simulink library "carnotUIBK"  (R2024b)
settings: Solver=VariableStepAuto  StartTime=0.0  StopTime=10.0  RelTol=1e-3  EnableMultiTasking=on
values from neighbouring files (symbols this model uses):
  area = area + room(kk).area    [THERMALZONE.m]
  boundary = BOUNDARY()    [BUILDING.m]
  building = obj    [BUILDING.m]
  C = zeros(1,length(d)+1)    [CONSTRUCTION.m]
  cp = str2num(value)    [CONSTRUCTION.m]
  pos = find(d_layer>0)    [CONSTRUCTION.m]
  rho = str2num(value)    [CONSTRUCTION.m]
  type = 1    [CONSTRUCTION.m]
  zone = obj.zone(ind)    [THERMALZONE.m]
undefined symbols (not defined in the file or in its folder): A, amb_factor, B, const, control, Dd, get_building, height, p, Qdot_C, Qdot_H, Qdot_I_electricity, Qdot_I_light, Qdot_I_person, Qdot_S, Qdot_T_ground, Qdot_T_neighbour, Qdot_T_opaque, Qdot_T_window, Qdot_V_infiltration, Qdot_V_mech, Qdot_V_window, r_frame, solar_ratio, solar_ratio1, solar_ratio2, Tc, Tr, Ts, Uvalue, view_factor, wall, wallsurface, window, window_height, window_heigth, window_width, windowsurface, x_CO2, x_H2O, x_VOC, z
libraries: carnot x105, $bdroot x22, simulink x18, simulink_extras x14
(part 3 of 13)

== system carnotUIBK/airexchange_intersection/EMPTY ==
  AIB1 : Inport
  AIB2 : Inport  Port=2
  control : Inport  Port=3
  Constant{,1..12,17..19} (16 alike) : Constant  Value=0
  Constant13 : Constant  Value=zeros(1,6)
  Constant14 : Constant  Value=zeros(1,5)
  Constant15 : Constant  Value=zeros(1,6)
  Constant16 : Constant  Value=zeros(1,5)
  Mux1 : Mux  Inputs=[1 1 1 1 1 1 1 6 1 5]
  Mux2 : Mux  Inputs=[1 1 1 1 1 1 1 6 1 5]
  Selector1 : Selector  InputPortWidth=NUMBEROFCONTROLS  IndexOptions=Index vector (dialog)  Indices=[control]  OutputSizes=1
  Terminator : Terminator
  Terminator1 : Terminator
  Terminator2 : Terminator
  "[S1]" : Outport  InitialOutput=0  VectorParamsAs1DForOutWhenUnconnected=off
  "[S2]" : Outport  Port=2  InitialOutput=0  VectorParamsAs1DForOutWhenUnconnected=off
  wires:
  Constant1/1 -> Mux1/4
  Constant4/1 -> Mux1/9
  Constant3/1 -> Mux1/6
  Constant2/1 -> Mux1/5
  Constant/1 -> Mux1/1
  Mux1/1 -> "[S1]"/1
  AIB2/1 -> Terminator2/1
  AIB1/1 -> Terminator1/1
  Constant11/1 -> Mux1/3
  Constant10/1 -> Mux1/2
  Constant12/1 -> Mux1/7
  Constant13/1 -> Mux1/8
  Constant14/1 -> Mux1/10
  control/1 -> Selector1/1
  Selector1/1 -> Terminator/1
  Mux2/1 -> "[S2]"/1
  Constant6/1 -> Mux2/4
  Constant19/1 -> Mux2/9
  Constant18/1 -> Mux2/6
  Constant17/1 -> Mux2/5
  Constant5/1 -> Mux2/1
  Constant8/1 -> Mux2/3
  Constant7/1 -> Mux2/2
  Constant9/1 -> Mux2/7
  Constant15/1 -> Mux2/8
  Constant16/1 -> Mux2/10

== system carnotUIBK/airexchange_intersection/airexchange_empiric ==
  note: ASSUMPTION: mdot_air_in = mdot_air_out !
  AIB1 : Inport
  AIB2 : Inport  Port=2
  control : Inport  Port=3
  1/3600 : Gain  Gain=1/3600
  Bus Selector1 : BusSelector  OutputSignals=Tc,x_H2O,x_CO2
  Bus Selector2 : BusSelector  OutputSignals=Tc,x_H2O,x_CO2,rho,cp
  Constant{4..6,9,15..16} (6 alike) : Constant  Value=0
  Constant17 : Constant  Value=zeros(1,2)
  Constant18 : Constant  Value=zeros(1,9)
  Constant7 : Constant  Value=zeros(1,2)
  Constant8 : Constant  Value=zeros(1,9)
  Gain{1,4..6} (4 alike) : Gain  Gain=-1
  Gain2 : Gain  Gain=0
  Gain3 : Gain  Gain=0
  Mux : Mux  Inputs=2
  Mux1 : Mux  Inputs=[1 1 1 1 1 1 1 2 1 9]
  Mux2 : Mux  Inputs=[1 1 1 1 1 1 1 2 1 9]
  Mux3 : Mux  Inputs=2
  Product2 : Product  InputSameDT=on  SaturateOnIntegerOverflow=on  OutDataTypeStr=Inherit: Same as first input
  Product4 : Product  Inputs=3  InputSameDT=on  SaturateOnIntegerOverflow=on  OutDataTypeStr=Inherit: Same as first input
  Selector1 : Selector  InputPortWidth=NUMBEROFCONTROLS  IndexOptions=Index vector (dialog)  Indices=[control]  OutputSizes=1
  Subsystem : Subsystem
  Sum : Sum  Inputs=-+  InputSameDT=on  SaturateOnIntegerOverflow=on  OutDataTypeStr=Inherit: Same as first input
  V exchange : Subsystem
  "[S1]" : Outport  InitialOutput=0  VectorParamsAs1DForOutWhenUnconnected=off
  "[S2]" : Outport  Port=2  InitialOutput=0  VectorParamsAs1DForOutWhenUnconnected=off
  wires:
  Gain2/1 -> Mux1/4
  Sum/1 -> Product4/1  "dT"
  Bus Selector2/5 -> Product4/2  "<cp>"
  Mux1/1 -> "[S1]"/1
  Bus Selector2/3 -> Mux/2  "<x_CO2>"
  control/1 -> Selector1/1
  AIB1/1 -> Bus Selector2/1
  AIB2/1 -> Bus Selector1/1
  Bus Selector2/4 -> Product2/2  "<rho>"
  Product4/1 -> Gain4/1, Gain1/1, Mux1/9, Mux1/1  "Qdot_air"
  Subsystem/2(mdot_CO2) -> Mux1/6, Gain6/1  "mdot_CO2"
  Subsystem/1(mdot_H2O) -> Gain5/1, Mux1/5  "mdot_H2O"
  Bus Selector2/2 -> V exchange/2(x in), Mux/1  "<x_H2O>"
  Mux/1 -> Subsystem/2(x_in)
  Mux3/1 -> Subsystem/3(x_out)
  Selector1/1 -> V exchange/5(control)
  Mux2/1 -> "[S2]"/1
  Bus Selector1/2 -> V exchange/4(x out), Mux3/1  "<x_H2O>"
  Bus Selector1/3 -> Mux3/2  "<x_CO2>"
  V exchange/1(V exchange) -> 1/3600/1
  Bus Selector1/1 -> Sum/2, V exchange/3(Tc out)  "<Tc>"
  Bus Selector2/1 -> Sum/1, V exchange/1(Tc in)  "<Tc>"
  1/3600/1 -> Product2/1
  Product2/1 -> Product4/3, Subsystem/1(mdot_air), Gain2/1, Gain3/1
  Constant5/1 -> Mux1/3
  Constant4/1 -> Mux1/2
  Constant6/1 -> Mux1/7
  Constant7/1 -> Mux1/8
  Constant8/1 -> Mux1/10
  Constant15/1 -> Mux2/3
  Constant9/1 -> Mux2/2
  Constant16/1 -> Mux2/7
  Constant17/1 -> Mux2/8
  Constant18/1 -> Mux2/10
  Gain1/1 -> Mux2/9
  Gain3/1 -> Mux2/4
  Gain4/1 -> Mux2/1
  Gain5/1 -> Mux2/5
  Gain6/1 -> Mux2/6

== system carnotUIBK/airexchange_intersection/airexchange_powerlaw ==
  note: ASSUMPTION: mdot_air_in = mdot_air_out !
  AIB1 : Inport
  AIB2 : Inport  Port=2
  control : Inport  Port=3
  Bus Selector2 : BusSelector  OutputSignals=Tc,x_H2O,x_CO2,rho
  Bus Selector3 : BusSelector  OutputSignals=Tc,x_H2O,x_CO2,rho,cp
  Constant{4..6,9,15..16} (6 alike) : Constant  Value=0
  Constant17 : Constant  Value=zeros(1,2)
  Constant18 : Constant  Value=zeros(1,9)
  Constant7 : Constant  Value=zeros(1,2)
  Constant8 : Constant  Value=zeros(1,9)
  Divide1 : Product  Inputs=*/
  Gain{1,4..6} (4 alike) : Gain  Gain=-1
  Gain2 : Gain  Gain=0
  Gain3 : Gain  Gain=0
  Mux : Mux  Inputs=2
  Mux1 : Mux  Inputs=[1 1 1 1 1 1 1 2 1 9]
  Mux2 : Mux  Inputs=[1 1 1 1 1 1 1 2 1 9]
  Mux3 : Mux  Inputs=2
  Product4 : Product  Inputs=3  InputSameDT=on  SaturateOnIntegerOverflow=on  OutDataTypeStr=Inherit: Same as first input
  Selector1 : Selector  InputPortWidth=NUMBEROFCONTROLS  IndexOptions=Index vector (dialog)  Indices=[control]  OutputSizes=1
  Subsystem : Subsystem
  Sum : Sum  Inputs=-+  InputSameDT=on  SaturateOnIntegerOverflow=on  OutDataTypeStr=Inherit: Same as first input
  Transfer Fcn : TransferFcn  Denominator=[100 1]
  door open : Subsystem
  "door_area " : Constant  Value=area
  door_height : Constant  Value=height
  "door_height " : Constant  Value=height
  "[S1]" : Outport  InitialOutput=0  VectorParamsAs1DForOutWhenUnconnected=off
  "[S2]" : Outport  Port=2  InitialOutput=0  VectorParamsAs1DForOutWhenUnconnected=off
  wires:
  Gain2/1 -> Mux1/4
  Sum/1 -> Product4/1  "dT"
  Bus Selector3/5 -> Product4/2  "<cp>"
  Mux1/1 -> "[S1]"/1
  Bus Selector3/3 -> Mux/2  "<x_CO2>"
  control/1 -> Selector1/1
  AIB1/1 -> Bus Selector3/1
  AIB2/1 -> Bus Selector2/1
  Bus Selector2/1 -> Sum/2  "<Tc>"
  Bus Selector3/2 -> Mux/1  "<x_H2O>"
  Mux/1 -> Subsystem/2(x_in)
  Bus Selector3/1 -> Sum/1  "<Tc>"
  Mux3/1 -> Subsystem/3(x_out)
  Selector1/1 -> door open/5(control)
  door open/1(m_dot_open_door) -> Transfer Fcn/1
  Mux2/1 -> "[S2]"/1
  Product4/1 -> Gain6/1, Gain1/1, Mux1/9, Mux1/1  "Qdot_air"
  Subsystem/2(mdot_CO2) -> Gain4/1, Mux1/6  "mdot_CO2"
  Subsystem/1(mdot_H2O) -> Gain5/1, Mux1/5  "mdot_H2O"
  Bus Selector2/2 -> Mux3/1  "<x_H2O>"
  Bus Selector2/3 -> Mux3/2  "<x_CO2>"
  door_height/1 -> door open/1(H (height of the door [m]))
  Divide1/1 -> door open/4(L)  "door width"
  Bus Selector3/4 -> door open/2(rho_i)  "<rho>"
  Bus Selector2/4 -> door open/3(rho_j)  "<rho>"
  "door_area "/1 -> Divide1/1
  "door_height "/1 -> Divide1/2
  Constant5/1 -> Mux1/3
  Constant4/1 -> Mux1/2
  Constant6/1 -> Mux1/7
  Constant7/1 -> Mux1/8
  Constant8/1 -> Mux1/10
  Constant15/1 -> Mux2/3
  Constant9/1 -> Mux2/2
  Constant16/1 -> Mux2/7
  Constant17/1 -> Mux2/8
  Constant18/1 -> Mux2/10
  Gain1/1 -> Mux2/9
  Gain3/1 -> Mux2/4
  Gain4/1 -> Mux2/6
  Gain5/1 -> Mux2/5
  Gain6/1 -> Mux2/1
  Transfer Fcn/1 -> Gain3/1, Gain2/1, Subsystem/1(mdot_air), Product4/3

== system carnotUIBK/boundary/GDB ==
  GDB_create : BusCreator  Inputs=6
  ground_1 : FromWorkspace  VariableName=b.boundary.ground(1).temperature
  ground_2 : FromWorkspace  VariableName=b.boundary.ground(2).temperature
  ground_3 : FromWorkspace  VariableName=b.boundary.ground(3).temperature
  ground_4 : FromWorkspace  VariableName=b.boundary.ground(4).temperature
  ground_5 : FromWorkspace  VariableName=b.boundary.ground(5).temperature
  ground_6 : FromWorkspace  VariableName=b.boundary.ground(6).temperature
  GDB : Outport  VectorParamsAs1DForOutWhenUnconnected=off
  wires:
  ground_1/1 -> GDB_create/1  "ground_1"
  ground_3/1 -> GDB_create/3  "ground_3"
  ground_2/1 -> GDB_create/2  "ground_2"
  ground_6/1 -> GDB_create/6  "ground_6"
  ground_4/1 -> GDB_create/4  "ground_4"
  GDB_create/1 -> GDB/1
  ground_5/1 -> GDB_create/5  "ground_5"

== system carnotUIBK/boundary/NDB ==
  GDB_create : BusCreator  Inputs=6
  neighbour_1 : FromWorkspace  VariableName=b.boundary.neighbour(1).temperature
  neighbour_2 : FromWorkspace  VariableName=b.boundary.neighbour(2).temperature
  neighbour_3 : FromWorkspace  VariableName=b.boundary.neighbour(3).temperature
  neighbour_4 : FromWorkspace  VariableName=b.boundary.neighbour(4).temperature
  neighbour_5 : FromWorkspace  VariableName=b.boundary.neighbour(5).temperature
  neighbour_6 : FromWorkspace  VariableName=b.boundary.neighbour(6).temperature
  NDB : Outport  VectorParamsAs1DForOutWhenUnconnected=off
  wires:
  neighbour_5/1 -> GDB_create/5  "neighbour_5"
  GDB_create/1 -> NDB/1
  neighbour_4/1 -> GDB_create/4  "neighbour_4"
  neighbour_6/1 -> GDB_create/6  "neighbour_6"
  neighbour_2/1 -> GDB_create/2  "neighbour_2"
  neighbour_3/1 -> GDB_create/3  "neighbour_3"
  neighbour_1/1 -> GDB_create/1  "neighbour_1"

== system carnotUIBK/boundary/WDB ==
  I_diffuse_surface : FromWorkspace  VariableName=we.Idiffuse_surface
  I_direct_surface : FromWorkspace  VariableName=we.Idirect_surface
  WDB_Creator : carnot/Basic/Weather_and_Sun/WDB_Creator
      settings: SourceProductName=Carnot
  azimuth : FromWorkspace  VariableName=we.azimuth
  cloud_index : FromWorkspace  VariableName=we.cloud
  incidence : FromWorkspace  VariableName=we.incidence
  precipitation : FromWorkspace  VariableName=we.precip
  pressure : FromWorkspace  VariableName=we.p
  radiation_beam_normal : FromWorkspace  VariableName=we.radiation_beam_normal
  radiation_diffuse_horizontal : FromWorkspace  VariableName=we.radiation_diffuse_horizontal
  relative_humidity : FromWorkspace  VariableName=we.rh
  t_amb : FromWorkspace  VariableName=we.t_ambient
  t_sky : FromWorkspace  VariableName=we.t_sky
  teta_p : FromWorkspace  VariableName=we.tetap
  teta_s : FromWorkspace  VariableName=we.tetas
  time_value : FromWorkspace  VariableName=we.time_value
  vw : FromWorkspace  VariableName=we.vw
  wdir : FromWorkspace  VariableName=we.wdir
  zenith : FromWorkspace  VariableName=we.zenith
  WDB : Outport  VectorParamsAs1DForOutWhenUnconnected=off
  wires:
  radiation_beam_normal/1 -> WDB_Creator/4  "I_beam_normal"
  azimuth/1 -> WDB_Creator/3  "azimuth"
  t_amb/1 -> WDB_Creator/6  "Tamb"
  radiation_diffuse_horizontal/1 -> WDB_Creator/5  "I_diffuse_horizontal"
  time_value/1 -> WDB_Creator/1  "time_value"
  zenith/1 -> WDB_Creator/2  "zenith"
  t_sky/1 -> WDB_Creator/7  "Tsky"
  teta_p/1 -> WDB_Creator/15  "longitudinal_angle"
  relative_humidity/1 -> WDB_Creator/8  "relative_humidity"
  precipitation/1 -> WDB_Creator/9  "precipitation"
  cloud_index/1 -> WDB_Creator/10  "cloud_index"
  I_diffuse_surface/1 -> WDB_Creator/18  "I_diffuse_surface"
  pressure/1 -> WDB_Creator/11  "pressure"
  wdir/1 -> WDB_Creator/13  "wind_direction"
  teta_s/1 -> WDB_Creator/16  "transversal_angle"
  I_direct_surface/1 -> WDB_Creator/17  "I_direct_surface"
  vw/1 -> WDB_Creator/12  "wind_speed"
  incidence/1 -> WDB_Creator/14  "incidence_angle"
  WDB_Creator/1 -> WDB/1

== system carnotUIBK/gain/EMPTY ==
  AIB : Inport
  control : Inport  Port=2
  Constant13 : Constant  Value=zeros(1,19)
  Mux1 : Mux  Inputs=[19]
  Selector1 : Selector  InputPortWidth=NUMBEROFCONTROLS  IndexOptions=Index vector (dialog)  Indices=[control]  OutputSizes=1
  Terminator : Terminator
  Terminator1 : Terminator
  "[S]" : Outport  VectorParamsAs1DForOutWhenUnconnected=off
  wires:
  AIB/1 -> Terminator/1
  Mux1/1 -> "[S]"/1
  control/1 -> Selector1/1
  Selector1/1 -> Terminator1/1
  Constant13/1 -> Mux1/1

== system carnotUIBK/gain/Equipment ==
  AIB : Inport
  control : Inport  Port=2
  0 : Constant  Value=0
  1 : Constant
  Product : Product
  Selector1 : Selector  InputPortWidth=NUMBEROFCONTROLS  IndexOptions=Index vector (dialog)  Indices=[control]  OutputSizes=1
  Sum : Sum  Inputs=|+-
  Sum1 : Sum  InputSameDT=on  SaturateOnIntegerOverflow=on  OutDataTypeStr=Inherit: Same as first input
  Sum2 : Sum  Inputs=|+-
  Switch : Constant  Value=type
  Switch1 : Switch  Criteria=u2 ~= 0  SaturateOnIntegerOverflow=off  InputSameDT=off
  Switch2 : Switch  Criteria=u2 ~= 0  SaturateOnIntegerOverflow=off  InputSameDT=off
  Terminator : Terminator
  W/device : Subsystem
  W/m² : Subsystem
  none : Constant  Value=0
  none1 : Constant  Value=0
  okay : Constant
  okay1 : Constant
  "[S]" : Outport  VectorParamsAs1DForOutWhenUnconnected=off
  wires:
  W/m²/1("[S]") -> Sum1/2
  W/device/1("[S]") -> Sum1/1
  Switch/1 -> Sum/1, Sum2/1
  0/1 -> Sum/2
  Sum/1 -> Switch1/2
  okay/1 -> Switch1/3
  none/1 -> Switch1/1
  1/1 -> Sum2/2
  Sum2/1 -> Switch2/2
  okay1/1 -> Switch2/3
  none1/1 -> Switch2/1
  Switch1/1 -> W/device/1(Switch)
  Switch2/1 -> W/m²/1(Switch)
  AIB/1 -> Terminator/1
  control/1 -> Selector1/1
  Selector1/1 -> Product/2
  Product/1 -> "[S]"/1
  Sum1/1 -> Product/1

== system carnotUIBK/gain/Light ==
  AIB : Inport
  control : Inport  Port=2
  0 : Constant  Value=0
  1 : Constant
  Product : Product
  Selector1 : Selector  InputPortWidth=NUMBEROFCONTROLS  IndexOptions=Index vector (dialog)  Indices=[control]  OutputSizes=1
  Sum : Sum  Inputs=|+-
  Sum1 : Sum  InputSameDT=on  SaturateOnIntegerOverflow=on  OutDataTypeStr=Inherit: Same as first input
  Sum2 : Sum  Inputs=|+-
  Switch : Constant  Value=type
  Switch1 : Switch  Criteria=u2 ~= 0  SaturateOnIntegerOverflow=off  InputSameDT=off
  Switch2 : Switch  Criteria=u2 ~= 0  SaturateOnIntegerOverflow=off  InputSameDT=off
  Terminator : Terminator
  W/light : Subsystem
  W/m² : Subsystem
  none : Constant  Value=0
  none1 : Constant  Value=0
  okay : Constant
  okay1 : Constant
  "[S]" : Outport  VectorParamsAs1DForOutWhenUnconnected=off
  wires:
  W/m²/1("[S]") -> Sum1/2
  W/light/1("[S]") -> Sum1/1
  AIB/1 -> Terminator/1
  ? -> ?
  Switch/1 -> Sum/1, Sum2/1
  0/1 -> Sum/2
  Sum/1 -> Switch1/2
  okay/1 -> Switch1/3
  none/1 -> Switch1/1
  1/1 -> Sum2/2
  Sum2/1 -> Switch2/2
  okay1/1 -> Switch2/3
  none1/1 -> Switch2/1
  Switch1/1 -> W/light/1(Switch)
  Switch2/1 -> W/m²/1(Switch)
  control/1 -> Selector1/1
  Selector1/1 -> Product/2
  Product/1 -> "[S]"/1
  Sum1/1 -> Product/1

== system carnotUIBK/gain/Moisture ==
  AIB : Inport
  control : Inport  Port=2
  Product : Product
  Selector1 : Selector  InputPortWidth=NUMBEROFCONTROLS  IndexOptions=Index vector (dialog)  Indices=[control]  OutputSizes=1
  Terminator : Terminator
  kg/s : Subsystem
  "[S]" : Outport  VectorParamsAs1DForOutWhenUnconnected=off
  wires:
  AIB/1 -> Terminator/1
  control/1 -> Selector1/1
  Selector1/1 -> Product/2
  Product/1 -> "[S]"/1
  kg/s/1("[S]") -> Product/1

== system carnotUIBK/gain/People ==
  AIB : Inport
  control : Inport  Port=2
  0 : Constant  Value=0
  1 : Constant
  2 : Constant  Value=2
  Bus Selector : BusSelector  OutputSignals=Ts
  Constant : Constant  Value=type
  Product : Product
  Selector1 : Selector  InputPortWidth=NUMBEROFCONTROLS  IndexOptions=Index vector (dialog)  Indices=[control]  OutputSizes=1
  Sum : Sum  Inputs=|+-
  Sum1 : Sum  Inputs=+++  InputSameDT=on  SaturateOnIntegerOverflow=on  OutDataTypeStr=Inherit: Same as first input
  Sum2 : Sum  Inputs=|+-
  Sum3 : Sum  Inputs=|+-
  Switch : Switch  Criteria=u2 ~= 0  SaturateOnIntegerOverflow=off  InputSameDT=off
  Switch1 : Switch  Criteria=u2 ~= 0  SaturateOnIntegerOverflow=off  InputSameDT=off
  Switch2 : Switch  Criteria=u2 ~= 0  SaturateOnIntegerOverflow=off  InputSameDT=off
  W/m² : Subsystem
  W/ppl (activity) : Subsystem
  W/ppl (constant) : Subsystem
  none : Constant  Value=0
  none1 : Constant  Value=0
  none2 : Constant  Value=0
  okay : Constant
  okay1 : Constant
  okay2 : Constant
  "[S]" : Outport  VectorParamsAs1DForOutWhenUnconnected=off
  wires:
  W/m²/1("[S]") -> Sum1/3
  W/ppl (constant)/1("[S]") -> Sum1/1
  W/ppl (activity)/1("[S]") -> Sum1/2
  Constant/1 -> Sum/1, Sum2/1, Sum3/1
  0/1 -> Sum/2
  Sum/1 -> Switch/2
  okay/1 -> Switch/3
  none/1 -> Switch/1
  Switch/1 -> W/ppl (constant)/2(Switch)
  1/1 -> Sum2/2
  Sum2/1 -> Switch1/2
  Sum3/1 -> Switch2/2
  2/1 -> Sum3/2
  Switch1/1 -> W/ppl (activity)/2(Switch)
  Switch2/1 -> W/m²/1(Switch)
  okay1/1 -> Switch1/3
  none1/1 -> Switch1/1
  okay2/1 -> Switch2/3
  none2/1 -> Switch2/1
  AIB/1 -> Bus Selector/1
  Bus Selector/1 -> W/ppl (activity)/1(Top), W/ppl (constant)/1(Top)  "<Ts>"
  control/1 -> Selector1/1
  Selector1/1 -> Product/2
  Product/1 -> "[S]"/1
  Sum1/1 -> Product/1

== system carnotUIBK/general/S_initialize ==
  Bus Creator2 : BusCreator  Inputs=19
  Constant{,1..18} (19 alike) : Constant  Value=0
  S : Outport  VectorParamsAs1DForOutWhenUnconnected=off
  wires:
  Constant7/1 -> Bus Creator2/15  "Qdot_I_person"
  Constant11/1 -> Bus Creator2/18  "Qdot_H"
  Constant10/1 -> Bus Creator2/17  "Qdot_I_electricity"
  Constant9/1 -> Bus Creator2/16  "Qdot_I_light"
  Constant12/1 -> Bus Creator2/19  "Qdot_C"
  Bus Creator2/1 -> S/1
  Constant1/1 -> Bus Creator2/2  "Qdotr"
  Constant/1 -> Bus Creator2/1  "Qdotc"
  Constant8/1 -> Bus Creator2/3  "Qdot_S"
  Constant14/1 -> Bus Creator2/5  "mdot_H2O"
  Constant13/1 -> Bus Creator2/4  "mdot_air"
  Constant15/1 -> Bus Creator2/6  "mdot_CO2"
  Constant16/1 -> Bus Creator2/7  "mdot_VOC"
  Constant17/1 -> Bus Creator2/8  "Qdot_T_opaque"
  Constant5/1 -> Bus Creator2/13  "Qdot_V_window"
  Constant4/1 -> Bus Creator2/12  "Qdot_V_mech"
  Constant2/1 -> Bus Creator2/10  "Qdot_T_neighbour"
  Constant6/1 -> Bus Creator2/14  "Qdot_V_infiltration"
  Constant3/1 -> Bus Creator2/11  "Qdot_T_window"
  Constant18/1 -> Bus Creator2/9  "Qdot_T_ground"

== system carnotUIBK/general/density and capacity ==
  T : Inport
  p : Inport  Port=2
  Add : Sum  Inputs=2
  Constant1 : Constant  Value=10000
  Constant2 : Constant  Value=0.0001
  Divide : Product  Inputs=*/
  K : Constant  Value=273.15
  Product : Product
  Product1 : Product
  Ra : Gain  Gain=287.058
  Rounding Function : Rounding
  cp_const : Constant  Value=1006.8
  rho : Outport  VectorParamsAs1DForOutWhenUnconnected=off
  cp : Outport  Port=2  VectorParamsAs1DForOutWhenUnconnected=off
  wires:
  Product1/1 -> rho/1
  Constant2/1 -> Product1/2
  Constant1/1 -> Product/2
  Product/1 -> Rounding Function/1
  Divide/1 -> Product/1
  Rounding Function/1 -> Product1/1
  Ra/1 -> Divide/2
  Add/1 -> Ra/1
  K/1 -> Add/2
  T/1 -> Add/1
  p/1 -> Divide/1
  cp_const/1 -> cp/1

== system carnotUIBK/infiltration/EMPTY ==
  AIB : Inport
  WDB : Inport  Port=2
  control : Inport  Port=3
  Constant{,1..4,10..12} (8 alike) : Constant  Value=0
  Constant13 : Constant  Value=zeros(1,6)
  Constant14 : Constant  Value=zeros(1,5)
  Mux1 : Mux  Inputs=[1 1 1 1 1 1 1 6 1 5]
  Selector1 : Selector  InputPortWidth=NUMBEROFCONTROLS  IndexOptions=Index vector (dialog)  Indices=[control]  OutputSizes=1
  Terminator : Terminator
  Terminator1 : Terminator
  Terminator2 : Terminator
  "[S]" : Outport  InitialOutput=0  VectorParamsAs1DForOutWhenUnconnected=off
  wires:
  Selector1/1 -> Terminator/1
  control/1 -> Selector1/1
  AIB/1 -> Terminator1/1
  WDB/1 -> Terminator2/1
  Mux1/1 -> "[S]"/1
  Constant1/1 -> Mux1/4
  Constant4/1 -> Mux1/9
  Constant3/1 -> Mux1/6
  Constant2/1 -> Mux1/5
  Constant/1 -> Mux1/1
  Constant11/1 -> Mux1/3
  Constant10/1 -> Mux1/2
  Constant12/1 -> Mux1/7
  Constant13/1 -> Mux1/8
  Constant14/1 -> Mux1/10

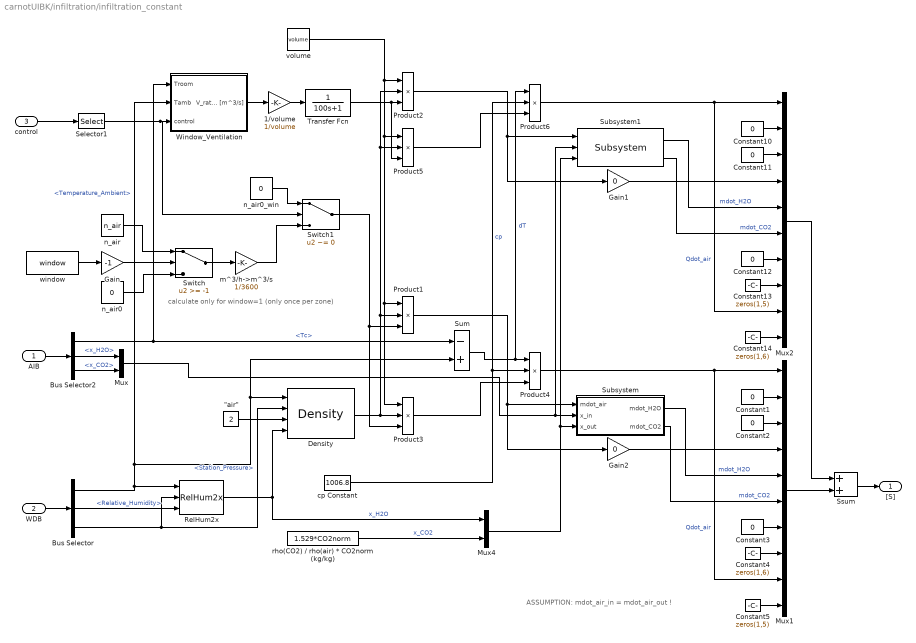
== system carnotUIBK/infiltration/infiltration_constant ==
  note: calculate only for window=1 (only once per zone)
  note: ASSUMPTION: mdot_air_in = mdot_air_out !
  AIB : Inport
  WDB : Inport  Port=2
  control : Inport  Port=3
  "\"air\"" : Constant  Value=2
  1/volume : Gain  Gain=1/volume
  Bus Selector : BusSelector  OutputSignals=Temperature_Ambient,Relative_Humidity,Station_Pressure
  Bus Selector2 : BusSelector  OutputSignals=Tc,x_H2O,x_CO2
  Constant{1..3,10..12} (6 alike) : Constant  Value=0
  Constant13 : Constant  Value=zeros(1,5)
  Constant14 : Constant  Value=zeros(1,6)
  Constant4 : Constant  Value=zeros(1,6)
  Constant5 : Constant  Value=zeros(1,5)
  Density : carnot/Basic/Material_Properties/Density  VariantControl=CarlibClassic  INPUTARGUMENTS=state variables (classic)  DEBUGLEVEL=NOLEVEL  MAXTOTALWARNINGS=inf  MAXCONSECUTIVEWARNINGS=inf  WRITETOFILE=0  FILENAME='errors.txt'
      settings: SourceProductName=Carnot
  Gain : Gain  Gain=-1
  Gain1 : Gain  Gain=0
  Gain2 : Gain  Gain=0
  Mux : Mux  Inputs=2
  Mux1 : Mux  Inputs=[1 1 1 1 1 1 1 6 1 5]
  Mux2 : Mux  Inputs=[1 1 1 1 1 1 1 5 1 6]
  Mux4 : Mux  Inputs=2
  Product{1..6} (6 alike) : Product  Inputs=3  InputSameDT=on  SaturateOnIntegerOverflow=on  OutDataTypeStr=Inherit: Same as first input
  RelHum2x : carnot/Basic/Material_Properties/RelHum2x
      settings: SourceProductName=Carnot
  Selector1 : Selector  InputPortWidth=NUMBEROFCONTROLS  IndexOptions=Index vector (dialog)  Indices=[control]  OutputSizes=1
  Ssum : Sum
  Subsystem : Subsystem
  Subsystem1 : $bdroot/infiltration/infiltration_constant/Subsystem  SystemSampleTime=-1  Latency=0  AutoFrameSizeCalculation=off
  Sum : Sum  Inputs=-+  InputSameDT=on  SaturateOnIntegerOverflow=on  OutDataTypeStr=Inherit: Same as first input
  Switch : Switch  Threshold=-1  SaturateOnIntegerOverflow=off  InputSameDT=off
  Switch1 : Switch  Criteria=u2 ~= 0  Threshold=-1  SaturateOnIntegerOverflow=off  InputSameDT=off
  Transfer Fcn : TransferFcn  Denominator=[100 1]
  Window_Ventilation : Subsystem  mask(window ventilation){alpha=10, H=window_width, W=window_height}
      mask prompts: alpha "maximal opening angle (°)"; H "height of window (m)"; W "width of window (m)"
      mask help: Simulates the free driven ventilation through a window with an opening angle of [0,1]* max. angle. Valid for angles between 8° and 180°. Output is the VOLUME FLOW RATE in m^3/s. Calculation based on the Ansatz from Weber.
      mask Display: plot(0,10,90,80,[20 70 70 20 20],[20 20 70 70 20],[20 70 80 30 20],[20 20 65 65 20])
  cp Constant : Constant  Value=1006.8
  m^3/h->m^3/s : Gain  Gain=1/3600
  n_air : Constant  Value=n_air
  n_air0 : Constant  Value=0
  n_air0_win : Constant  Value=0
  rho(CO2) / rho(air) * CO2norm (kg/kg) : Constant  Value=1.529*CO2norm
  volume : Constant  Value=volume
  window : Constant  Value=window
  "[S]" : Outport  InitialOutput=0  VectorParamsAs1DForOutWhenUnconnected=off
  wires:
  rho(CO2) / rho(air) * CO2norm (kg/kg)/1 -> Mux4/2  "x_CO2"
  Mux4/1 -> Subsystem1/3, Subsystem/3(x_out)
  Bus Selector2/1 -> Window_Ventilation/1(Troom), Sum/1  "<Tc>"
  Mux/1 -> Subsystem1/2, Subsystem/2(x_in)
  "\"air\""/1 -> Density/3
  RelHum2x/1 -> Density/4, Mux4/1  "x_H2O"
  Bus Selector/1 -> RelHum2x/1, Density/1, Sum/2, Window_Ventilation/2(Tamb)  "<Temperature_Ambient>"
  Bus Selector/2 -> RelHum2x/3  "<Relative_Humidity>"
  Bus Selector/3 -> Density/2, RelHum2x/2  "<Station_Pressure>"
  Subsystem/1(mdot_H2O) -> Mux1/5  "mdot_H2O"
  Subsystem/2(mdot_CO2) -> Mux1/6  "mdot_CO2"
  Product4/1 -> Mux1/9, Mux1/1  "Qdot_air"
  volume/1 -> Product1/1, Product3/1, Product5/1, Product2/1
  Product3/1 -> Product4/3
  Product1/1 -> Gain2/1, Subsystem/1(mdot_air)
  Density/1 -> Product3/2, Product2/2, Product5/2, Product1/2
  Switch/1 -> m^3/h->m^3/s/1
  WDB/1 -> Bus Selector/1
  AIB/1 -> Bus Selector2/1
  control/1 -> Selector1/1
  Selector1/1 -> Switch1/2, Window_Ventilation/3(control)
  n_air/1 -> Switch/1
  n_air0/1 -> Switch/3
  window/1 -> Gain/1
  Gain/1 -> Switch/2
  Window_Ventilation/1(V_rate [m^3/s]) -> 1/volume/1
  Switch1/1 -> Product3/3, Product1/3
  1/volume/1 -> Transfer Fcn/1
  Bus Selector2/2 -> Mux/1  "<x_H2O>"
  Bus Selector2/3 -> Mux/2  "<x_CO2>"
  Mux1/1 -> Ssum/2
  Ssum/1 -> "[S]"/1
  cp Constant/1 -> Product6/2, Product4/2  "cp"
  Sum/1 -> Product6/1, Product4/1  "dT"
  Subsystem1/1 -> Mux2/5  "mdot_H2O"
  Subsystem1/2 -> Mux2/6  "mdot_CO2"
  Product6/1 -> Mux2/1, Mux2/9  "Qdot_air"
  Product5/1 -> Product6/3
  Product2/1 -> Subsystem1/1, Gain1/1
  Mux2/1 -> Ssum/1
  m^3/h->m^3/s/1 -> Switch1/3
  n_air0_win/1 -> Switch1/1
  Gain1/1 -> Mux2/4
  Gain2/1 -> Mux1/4
  Constant11/1 -> Mux2/3
  Constant10/1 -> Mux2/2
  Constant12/1 -> Mux2/7
  Constant13/1 -> Mux2/8
  Constant14/1 -> Mux2/10
  Constant2/1 -> Mux1/3
  Constant1/1 -> Mux1/2
  Constant3/1 -> Mux1/7
  Constant4/1 -> Mux1/8
  Constant5/1 -> Mux1/10
  Transfer Fcn/1 -> Product5/3, Product2/3

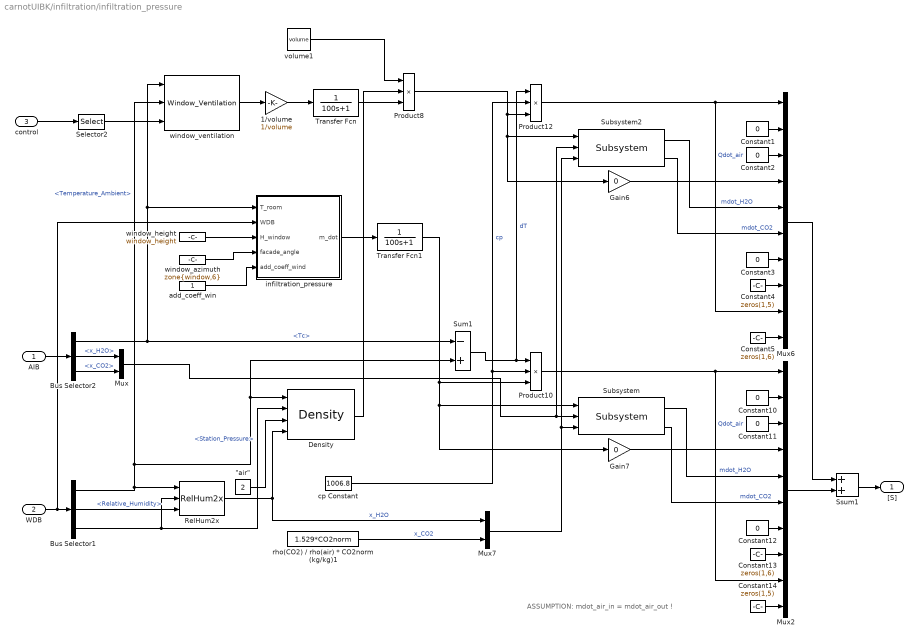
== system carnotUIBK/infiltration/infiltration_pressure ==
  note: ASSUMPTION: mdot_air_in = mdot_air_out !
  AIB : Inport
  WDB : Inport  Port=2
  control : Inport  Port=3
  "\"air\"" : Constant  Value=2
  1/volume : Gain  Gain=1/volume
  Bus Selector1 : BusSelector  OutputSignals=Temperature_Ambient,Relative_Humidity,Station_Pressure
  Bus Selector2 : BusSelector  OutputSignals=Tc,x_H2O,x_CO2
  Constant{1..3,10..12} (6 alike) : Constant  Value=0
  Constant13 : Constant  Value=zeros(1,6)
  Constant14 : Constant  Value=zeros(1,5)
  Constant4 : Constant  Value=zeros(1,5)
  Constant5 : Constant  Value=zeros(1,6)
  Density : carnot/Basic/Material_Properties/Density  VariantControl=CarlibClassic  INPUTARGUMENTS=state variables (classic)  DEBUGLEVEL=NOLEVEL  MAXTOTALWARNINGS=inf  MAXCONSECUTIVEWARNINGS=inf  WRITETOFILE=0  FILENAME='errors.txt'
      settings: SourceProductName=Carnot
  Gain6 : Gain  Gain=0
  Gain7 : Gain  Gain=0
  Mux : Mux  Inputs=2
  Mux2 : Mux  Inputs=[1 1 1 1 1 1 1 6 1 5]
  Mux6 : Mux  Inputs=[1 1 1 1 1 1 1 5 1 6]
  Mux7 : Mux  Inputs=2
  Product10 : Product  Inputs=3  InputSameDT=on  SaturateOnIntegerOverflow=on  OutDataTypeStr=Inherit: Same as first input
  Product12 : Product  Inputs=3  InputSameDT=on  SaturateOnIntegerOverflow=on  OutDataTypeStr=Inherit: Same as first input
  Product8 : Product  Inputs=3  InputSameDT=on  SaturateOnIntegerOverflow=on  OutDataTypeStr=Inherit: Same as first input
  RelHum2x : carnot/Basic/Material_Properties/RelHum2x
      settings: SourceProductName=Carnot
  Selector2 : Selector  InputPortWidth=NUMBEROFCONTROLS  IndexOptions=Index vector (dialog)  Indices=[control]  OutputSizes=1
  Ssum1 : Sum
  Subsystem : $bdroot/infiltration/infiltration_constant/Subsystem  SystemSampleTime=-1  Latency=0  AutoFrameSizeCalculation=off
  Subsystem2 : $bdroot/infiltration/infiltration_constant/Subsystem  SystemSampleTime=-1  Latency=0  AutoFrameSizeCalculation=off
  Sum1 : Sum  Inputs=-+  InputSameDT=on  SaturateOnIntegerOverflow=on  OutDataTypeStr=Inherit: Same as first input
  Transfer Fcn : TransferFcn  Denominator=[100 1]
  Transfer Fcn1 : TransferFcn  Denominator=[100 1]
  add_coeff_win : Constant
  cp Constant : Constant  Value=1006.8
  infiltration_pressure : Subsystem
  rho(CO2) / rho(air) * CO2norm (kg/kg)1 : Constant  Value=1.529*CO2norm
  volume1 : Constant  Value=volume
  window_azimuth : Constant  Value=zone{window,6}
  window_height : Constant  Value=window_height
  window_ventilation : $bdroot/infiltration/infiltration_constant/Window_Ventilation  alpha=10  H=window_width  W=window_height
  "[S]" : Outport  InitialOutput=0  VectorParamsAs1DForOutWhenUnconnected=off
  wires:
  rho(CO2) / rho(air) * CO2norm (kg/kg)1/1 -> Mux7/2  "x_CO2"
  Mux7/1 -> Subsystem2/3, Subsystem/3
  Mux/1 -> Subsystem2/2, Subsystem/2
  "\"air\""/1 -> Density/3
  RelHum2x/1 -> Density/4, Mux7/1  "x_H2O"
  Bus Selector1/1 -> RelHum2x/1, Density/1, Sum1/2, window_ventilation/2  "<Temperature_Ambient>"
  Bus Selector1/2 -> RelHum2x/3  "<Relative_Humidity>"
  Bus Selector1/3 -> Density/2, RelHum2x/2  "<Station_Pressure>"
  Subsystem/1 -> Mux2/5  "mdot_H2O"
  Subsystem/2 -> Mux2/6  "mdot_CO2"
  Product10/1 -> Mux2/9, Mux2/1  "Qdot_air"
  volume1/1 -> Product8/1
  Density/1 -> Product8/2
  AIB/1 -> Bus Selector2/1
  control/1 -> Selector2/1
  Selector2/1 -> window_ventilation/3
  window_ventilation/1 -> 1/volume/1
  1/volume/1 -> Transfer Fcn/1
  Bus Selector2/2 -> Mux/1  "<x_H2O>"
  Bus Selector2/3 -> Mux/2  "<x_CO2>"
  Mux2/1 -> Ssum1/2
  Ssum1/1 -> "[S]"/1
  cp Constant/1 -> Product12/2, Product10/2  "cp"
  Sum1/1 -> Product12/1, Product10/1  "dT"
  Subsystem2/1 -> Mux6/5  "mdot_H2O"
  Subsystem2/2 -> Mux6/6  "mdot_CO2"
  Product12/1 -> Mux6/1, Mux6/9  "Qdot_air"
  Product8/1 -> Product12/3, Subsystem2/1, Gain6/1
  Mux6/1 -> Ssum1/1
  Gain6/1 -> Mux6/4
  Gain7/1 -> Mux2/4
  Bus Selector2/1 -> Sum1/1, infiltration_pressure/1(T_room), window_ventilation/1  "<Tc>"
  WDB/1 -> infiltration_pressure/2(WDB), Bus Selector1/1
  window_height/1 -> infiltration_pressure/3(H_window)
  window_azimuth/1 -> infiltration_pressure/4(facade_angle)
  add_coeff_win/1 -> infiltration_pressure/5(add_coeff_wind)
  infiltration_pressure/1(m_dot) -> Transfer Fcn1/1
  Constant11/1 -> Mux2/3
  Constant10/1 -> Mux2/2
  Constant12/1 -> Mux2/7
  Constant13/1 -> Mux2/8
  Constant14/1 -> Mux2/10
  Constant2/1 -> Mux6/3
  Constant1/1 -> Mux6/2
  Constant3/1 -> Mux6/7
  Constant4/1 -> Mux6/8
  Constant5/1 -> Mux6/10
  Transfer Fcn/1 -> Product8/3
  Transfer Fcn1/1 -> Gain7/1, Subsystem/1, Product10/3

== system carnotUIBK/room_node/1-node ==
  note: 1-node model
  sum([S]) : Inport
  AIB_initialize : $bdroot/room_node/EMPTY/AIB_initialize  SystemSampleTime=-1  VariantActivationTime=update diagram  AllowFlexibleInterface=on  Latency=0  AutoFrameSizeCalculation=off
  BDB_initialize : $bdroot/room_node/EMPTY/BDB_initialize  SystemSampleTime=-1  VariantActivationTime=update diagram  AllowFlexibleInterface=on  Latency=0  AutoFrameSizeCalculation=off
  Bus Assignment : BusAssignment  AssignedSignals=Ts,Tc,Tr,x_H2O,x_CO2,x_VOC,rho,cp,p
  Bus Assignment1 : BusAssignment  AssignedSignals=Qdot_T_opaque,Qdot_T_ground,Qdot_T_neighbour,Qdot_T_window,Qdot_V_mech,Qdot_V_window,Qdot_V_infiltration,Qdot_S,Qdot_I_person,Qdot_I_light,Qdot_I_electricity,Qdot_H,Qdot_C
  Bus Selector : BusSelector  OutputSignals=Tc,p,x_H2O
  Demux2 : Demux  Outputs=19
      settings: DisplayOption=none
  Gain : Gain
  Gain1 : Gain
  Transfer Fcn : TransferFcn  Denominator=[1 1]
  density and capacity : $bdroot/room_node/2-node/density and capacity  SystemSampleTime=-1  VariantActivationTime=update diagram  AllowFlexibleInterface=on  Latency=0  AutoFrameSizeCalculation=off
  fluid_type : Constant  Value=2
  mass blalance : Subsystem
  pressure : Subsystem
  sensitive_node : Subsystem
  BDB : Outport  VectorParamsAs1DForOutWhenUnconnected=off
  AIB : Outport  Port=2  VectorParamsAs1DForOutWhenUnconnected=off
  Qdot_sol : Outport  Port=3  VectorParamsAs1DForOutWhenUnconnected=off
  wires:
  sensitive_node/1(Tc) -> Gain/1, Bus Assignment/2, Gain1/1  "Ts"
  Demux2/1 -> sensitive_node/1(Qdotc)  "Qdotc"
  pressure/1(p) -> Bus Assignment/10
  Demux2/4 -> pressure/1(mdot_air)  "mdot_air"
  mass blalance/3(x_VOC) -> Bus Assignment/7  "x_VOC"
  mass blalance/2(x_CO2) -> Bus Assignment/6  "x_CO2"
  mass blalance/1(x_H2O) -> Bus Assignment/5  "x_H2O"
  Demux2/7 -> mass blalance/3(mdot_VOC)  "mdot_VOC"
  Demux2/6 -> mass blalance/2(mdot_CO2)  "mdot_CO2"
  Demux2/5 -> mass blalance/1(mdot_H2O)  "mdot_H2O"
  fluid_type/1 -> density and capacity/3
  Bus Selector/3 -> density and capacity/4  "<x_H2O>"
  Bus Selector/2 -> density and capacity/2  "<p>"
  Bus Selector/1 -> density and capacity/1  "<Tc>"
  Bus Assignment/1 -> pressure/2(AIB), mass blalance/4(AIB), Bus Selector/1, AIB/1
  density and capacity/1 -> Bus Assignment/8  "rho"
  density and capacity/2 -> Bus Assignment/9  "cp"
  Demux2/2 -> sensitive_node/2(Qdotr)  "Qdotr"
  Demux2/3 -> Transfer Fcn/1  "Qdot_S"
  sum([S])/1 -> Demux2/1
  Gain/1 -> Bus Assignment/4  "Tr"
  Gain1/1 -> Bus Assignment/3  "Tc"
  Demux2/8 -> Bus Assignment1/2  "Qdot_T_opaque"
  Demux2/9 -> Bus Assignment1/3  "Qdot_T_ground"
  Demux2/10 -> Bus Assignment1/4  "Qdot_T_neighbour"
  Demux2/11 -> Bus Assignment1/5  "Qdot_T_window"
  Demux2/12 -> Bus Assignment1/6  "Qdot_V_mech"
  Demux2/13 -> Bus Assignment1/7  "Qdot_V_window"
  Demux2/14 -> Bus Assignment1/8  "Qdot_V_infiltration"
  Demux2/15 -> Bus Assignment1/10  "Qdot_I_person"
  Demux2/16 -> Bus Assignment1/11  "Qdot_I_light"
  Demux2/17 -> Bus Assignment1/12  "Qdot_I_electricity"
  Demux2/18 -> Bus Assignment1/13  "Qdot_H"
  Demux2/19 -> Bus Assignment1/14  "Qdot_C"
  AIB_initialize/1 -> Bus Assignment/1
  BDB_initialize/1 -> Bus Assignment1/1
  Bus Assignment1/1 -> BDB/1
  Transfer Fcn/1 -> Qdot_sol/1, Bus Assignment1/9

== system carnotUIBK/room_node/1-node_womass ==
  note: 1-node model without mass balance
  sum([S]) : Inport
  AIB_initialize : $bdroot/room_node/EMPTY/AIB_initialize  SystemSampleTime=-1  VariantActivationTime=update diagram  AllowFlexibleInterface=on  Latency=0  AutoFrameSizeCalculation=off
  BDB_initialize : $bdroot/room_node/EMPTY/BDB_initialize  SystemSampleTime=-1  VariantActivationTime=update diagram  AllowFlexibleInterface=on  Latency=0  AutoFrameSizeCalculation=off
  Bus Assignment : BusAssignment  AssignedSignals=Ts,Tc,Tr,x_H2O,x_CO2,x_VOC,rho,cp,p
  Bus Assignment1 : BusAssignment  AssignedSignals=Qdot_T_opaque,Qdot_T_ground,Qdot_T_neighbour,Qdot_T_window,Qdot_V_mech,Qdot_V_window,Qdot_V_infiltration,Qdot_S,Qdot_I_person,Qdot_I_light,Qdot_I_electricity,Qdot_H,Qdot_C
  Demux2 : Demux  Outputs=19
      settings: DisplayOption=none
  Gain : Gain
  Gain1 : Gain
  Terminator{,1..3} (4 alike) : Terminator
  Transfer Fcn : TransferFcn  Denominator=[1 1]
  cp : Constant  Value=1.0068e3
  cp1 : Constant  Value=1e5
  rho : Constant  Value=1.1893
  sensitive_node : Subsystem
  x_CO2 : Constant  Value=0
  x_H2O : Constant  Value=0
  x_VOC : Constant  Value=0
  BDB : Outport  VectorParamsAs1DForOutWhenUnconnected=off
  AIB : Outport  Port=2  VectorParamsAs1DForOutWhenUnconnected=off
  Qdot_sol : Outport  Port=3  VectorParamsAs1DForOutWhenUnconnected=off
  wires:
  sensitive_node/1(Tc) -> Gain/1, Bus Assignment/2, Gain1/1  "Ts"
  Demux2/1 -> sensitive_node/1(Qdotc)  "Qdotc"
  cp1/1 -> Bus Assignment/10  "p"
  Demux2/4 -> Terminator/1  "mdot_air"
  x_VOC/1 -> Bus Assignment/7  "x_VOC"
  x_CO2/1 -> Bus Assignment/6  "x_CO2"
  x_H2O/1 -> Bus Assignment/5  "x_H2O"
  Demux2/7 -> Terminator3/1  "mdot_VOC"
  Demux2/6 -> Terminator2/1  "mdot_CO2"
  Demux2/5 -> Terminator1/1  "mdot_H2O"
  Bus Assignment/1 -> AIB/1
  rho/1 -> Bus Assignment/8  "rho"
  cp/1 -> Bus Assignment/9  "cp"
  Demux2/2 -> sensitive_node/2(Qdotr)  "Qdotr"
  Demux2/3 -> Transfer Fcn/1  "Qdot_S"
  sum([S])/1 -> Demux2/1
  Gain/1 -> Bus Assignment/4  "Tr"
  Gain1/1 -> Bus Assignment/3  "Tc"
  Demux2/8 -> Bus Assignment1/2  "Qdot_T_opaque"
  Demux2/9 -> Bus Assignment1/3  "Qdot_T_ground"
  Demux2/10 -> Bus Assignment1/4  "Qdot_T_neighbour"
  Demux2/11 -> Bus Assignment1/5  "Qdot_T_window"
  Demux2/12 -> Bus Assignment1/6  "Qdot_V_mech"
  Demux2/13 -> Bus Assignment1/7  "Qdot_V_window"
  Demux2/14 -> Bus Assignment1/8  "Qdot_V_infiltration"
  Demux2/15 -> Bus Assignment1/10  "Qdot_I_person"
  Demux2/16 -> Bus Assignment1/11  "Qdot_I_light"
  Demux2/17 -> Bus Assignment1/12  "Qdot_I_electricity"
  Demux2/18 -> Bus Assignment1/13  "Qdot_H"
  Demux2/19 -> Bus Assignment1/14  "Qdot_C"
  AIB_initialize/1 -> Bus Assignment/1
  BDB_initialize/1 -> Bus Assignment1/1
  Bus Assignment1/1 -> BDB/1
  Transfer Fcn/1 -> Qdot_sol/1, Bus Assignment1/9

== system carnotUIBK/room_node/2-node ==
  note: 2-node model
  sum([S]) : Inport
  AIB_initialize : $bdroot/room_node/EMPTY/AIB_initialize  SystemSampleTime=-1  VariantActivationTime=update diagram  AllowFlexibleInterface=on  Latency=0  AutoFrameSizeCalculation=off
  BDB_initialize : $bdroot/room_node/EMPTY/BDB_initialize  SystemSampleTime=-1  VariantActivationTime=update diagram  AllowFlexibleInterface=on  Latency=0  AutoFrameSizeCalculation=off
  Bus Assignment : BusAssignment  AssignedSignals=Ts,Tc,Tr,x_H2O,x_CO2,x_VOC,rho,cp,p
  Bus Assignment1 : BusAssignment  AssignedSignals=Qdot_T_opaque,Qdot_T_ground,Qdot_T_neighbour,Qdot_T_window,Qdot_V_mech,Qdot_V_window,Qdot_V_infiltration,Qdot_S,Qdot_I_person,Qdot_I_light,Qdot_I_electricity,Qdot_H,Qdot_C
  Bus Selector : BusSelector  OutputSignals=Tc,p,x_H2O
  Demux2 : Demux  Outputs=19
      settings: DisplayOption=none
  Sensitive room temperature : Subsystem  mask(SENSITIVE TEMPERATURE){share_c=50}
      mask prompts: share_c "SHARE of convective part, [0,100%]:"
      mask help:
      | This block merges the convective and radiative zone node temperature to the SENSITIVE ZONE TEMPERATURE (weighted arithmetic average of both components).
      |
      | [T] = [Tc; Tr]:  temperature vector of node, °C
      | Ts:              sensitive zone temperature, °C
      mask init:
      | blockname = gcb;
      | 
      | if (length(share_c)~=1) error(['PARAMETERS block "' blockname ': "SHARE of ..." must have only 1 entry !']); end;
      | if (share_c<0) | (share_c>100) error(['PARAMETERS block "' blockname '" : "SHARE of ..." must be within [0, 100%] !']); end;
      | share_c = share_c/100;
  convective_node : Subsystem
  density and capacity : Subsystem
  fluid_type : Constant  Value=2
  mass blalance : Subsystem
  pressure : Subsystem
  radiative_node : Subsystem
  BDB : Outport  VectorParamsAs1DForOutWhenUnconnected=off
  AIB : Outport  Port=2  VectorParamsAs1DForOutWhenUnconnected=off
  Qdot_sol : Outport  Port=3  VectorParamsAs1DForOutWhenUnconnected=off
  wires:
  radiative_node/1(Tr) -> Bus Assignment/4, Sensitive room temperature/1(Tr)  "Tr"
  Demux2/1 -> convective_node/1(Qdotc)  "Qdotc"
  pressure/1(p) -> Bus Assignment/10
  Demux2/4 -> pressure/1(mdot_air)  "mdot_air"
  mass blalance/3(x_VOC) -> Bus Assignment/7
  mass blalance/2(x_CO2) -> Bus Assignment/6
  mass blalance/1(x_H2O) -> Bus Assignment/5
  Demux2/7 -> mass blalance/3(mdot_VOC)  "mdot_VOC"
  Demux2/6 -> mass blalance/2(mdot_CO2)  "mdot_CO2"
  Demux2/5 -> mass blalance/1(mdot_H2O)  "mdot_H2O"
  fluid_type/1 -> density and capacity/3(fluid_type)
  Bus Selector/3 -> density and capacity/4(fluid_mix)  "<x_H2O>"
  Bus Selector/2 -> density and capacity/2(p)  "<p>"
  Bus Selector/1 -> density and capacity/1(T)  "<Tc>"
  Bus Assignment/1 -> convective_node/2(AIB), Bus Selector/1, mass blalance/4(AIB), pressure/2(AIB), AIB/1
  Sensitive room temperature/1(Ts) -> Bus Assignment/2  "Ts"
  convective_node/1(Tc) -> Bus Assignment/3, Sensitive room temperature/2(Tc)  "Tc"
  density and capacity/1(rho) -> Bus Assignment/8  "rho"
  density and capacity/2(cp) -> Bus Assignment/9  "cp"
  Demux2/2 -> radiative_node/1(Qdotr)  "Qdotr"
  Demux2/3 -> Qdot_sol/1, Bus Assignment1/9  "Qdot_S"
  sum([S])/1 -> Demux2/1
  Demux2/8 -> Bus Assignment1/2  "Qdot_T_opaque"
  Demux2/9 -> Bus Assignment1/3  "Qdot_T_ground"
  Demux2/10 -> Bus Assignment1/4  "Qdot_T_neighbour"
  Demux2/11 -> Bus Assignment1/5  "Qdot_T_window"
  Demux2/12 -> Bus Assignment1/6  "Qdot_V_mech"
  Demux2/13 -> Bus Assignment1/7  "Qdot_V_window"
  Demux2/14 -> Bus Assignment1/8  "Qdot_V_infiltration"
  Demux2/15 -> Bus Assignment1/10  "Qdot_I_person"
  Demux2/16 -> Bus Assignment1/11  "Qdot_I_light"
  Demux2/17 -> Bus Assignment1/12  "Qdot_I_electricity"
  Demux2/18 -> Bus Assignment1/13  "Qdot_H"
  Demux2/19 -> Bus Assignment1/14  "Qdot_C"
  AIB_initialize/1 -> Bus Assignment/1
  BDB_initialize/1 -> Bus Assignment1/1
  Bus Assignment1/1 -> BDB/1

== system carnotUIBK/room_node/2-node_ideal ==
  note: 2-node model ideal heating
  sum([S]) : Inport
  AIB_initialize : $bdroot/room_node/EMPTY/AIB_initialize  SystemSampleTime=-1  Latency=0  AutoFrameSizeCalculation=off
  BDB_initialize : $bdroot/room_node/EMPTY/BDB_initialize  SystemSampleTime=-1  Latency=0  AutoFrameSizeCalculation=off
  Bus Assignment : BusAssignment  AssignedSignals=Ts,Tc,Tr,x_H2O,x_CO2,x_VOC,rho,cp,p
  Bus Assignment1 : BusAssignment  AssignedSignals=Qdot_T_opaque,Qdot_T_ground,Qdot_T_neighbour,Qdot_T_window,Qdot_V_mech,Qdot_V_window,Qdot_V_infiltration,Qdot_S,Qdot_I_person,Qdot_I_light,Qdot_I_electricity,Qdot_H,Qdot_C
  Bus Selector : BusSelector  OutputSignals=Tc,p,x_H2O
  Compare To Zero : simulink/Logic and Bit Operations/Compare To Zero  relop=<=  OutDataTypeStr=boolean
  Compare To Zero1 : simulink/Logic and Bit Operations/Compare To Zero  relop=>=  OutDataTypeStr=boolean
  Demux2 : Demux  Outputs=19
      settings: DisplayOption=none
  Product : Product
  Product1 : Product
  Sensitive room temperature : Subsystem  mask(SENSITIVE TEMPERATURE){share_c=50}
      mask prompts: share_c "SHARE of convective part, [0,100%]:"
      mask help:
      | This block merges the convective and radiative zone node temperature to the SENSITIVE ZONE TEMPERATURE (weighted arithmetic average of both components).
      |
      | [T] = [Tc; Tr]:  temperature vector of node, °C
      | Ts:              sensitive zone temperature, °C
      mask init: same as carnotUIBK/room_node/2-node/Sensitive room temperature
  Tc : carnot/Load/General/Repeating_Profile  period=temperature_timevalues(end)  rep_seq_t=temperature_timevalues(1:end-1)  rep_seq_d=temperature_timeduration  rep_seq_y=temperature_Tc
      settings: SourceProductName=Carnot
  Tr : carnot/Load/General/Repeating_Profile  period=temperature_timevalues(end)  rep_seq_t=temperature_timevalues(1:end-1)  rep_seq_d=temperature_timeduration  rep_seq_y=temperature_Tr
      settings: SourceProductName=Carnot
  density and capacity : $bdroot/room_node/2-node/density and capacity  SystemSampleTime=-1  Latency=0  AutoFrameSizeCalculation=off
  fluid_type : Constant  Value=2
  heating : Sum  Inputs=--++
  mass blalance : Subsystem
  pressure : Subsystem
  BDB : Outport  VectorParamsAs1DForOutWhenUnconnected=off
  AIB : Outport  Port=2  VectorParamsAs1DForOutWhenUnconnected=off
  Qdot_sol : Outport  Port=3  VectorParamsAs1DForOutWhenUnconnected=off
  wires:
  Tr/1 -> Bus Assignment/4, Sensitive room temperature/1(Tr)  "Tr"
  Demux2/1 -> heating/1  "Qdotc"
  pressure/1(p) -> Bus Assignment/10
  Demux2/4 -> pressure/1(mdot_air)  "mdot_air"
  mass blalance/3(x_VOC) -> Bus Assignment/7
  mass blalance/2(x_CO2) -> Bus Assignment/6
  mass blalance/1(x_H2O) -> Bus Assignment/5
  Demux2/7 -> mass blalance/3(mdot_VOC)  "mdot_VOC"
  Demux2/6 -> mass blalance/2(mdot_CO2)  "mdot_CO2"
  Demux2/5 -> mass blalance/1(mdot_H2O)  "mdot_H2O"
  fluid_type/1 -> density and capacity/3
  Bus Selector/3 -> density and capacity/4  "<x_H2O>"
  Bus Selector/2 -> density and capacity/2  "<p>"
  Bus Selector/1 -> density and capacity/1  "<Tc>"
  Bus Assignment/1 -> AIB/1, pressure/2(AIB), mass blalance/4(AIB), Bus Selector/1
  Sensitive room temperature/1(Ts) -> Bus Assignment/2  "Ts"
  Tc/1 -> Bus Assignment/3, Sensitive room temperature/2(Tc)  "Tc"
  density and capacity/1 -> Bus Assignment/8  "rho"
  density and capacity/2 -> Bus Assignment/9  "cp"
  Demux2/2 -> heating/2  "Qdotr"
  sum([S])/1 -> Demux2/1
  Demux2/3 -> Bus Assignment1/9, Qdot_sol/1  "Qdot_S"
  Demux2/8 -> Bus Assignment1/2  "Qdot_T_opaque"
  Demux2/9 -> Bus Assignment1/3  "Qdot_T_ground"
  Demux2/10 -> Bus Assignment1/4  "Qdot_T_neighbour"
  Demux2/11 -> Bus Assignment1/5  "Qdot_T_window"
  Demux2/12 -> Bus Assignment1/6  "Qdot_V_mech"
  Demux2/13 -> Bus Assignment1/7  "Qdot_V_window"
  Demux2/14 -> Bus Assignment1/8  "Qdot_V_infiltration"
  Demux2/15 -> Bus Assignment1/10  "Qdot_I_person"
  Demux2/16 -> Bus Assignment1/11  "Qdot_I_light"
  Demux2/17 -> Bus Assignment1/12  "Qdot_I_electricity"
  Demux2/19 -> heating/4  "Qdot_C"
  Demux2/18 -> heating/3  "Qdot_H"
  AIB_initialize/1 -> Bus Assignment/1
  BDB_initialize/1 -> Bus Assignment1/1
  Bus Assignment1/1 -> BDB/1
  Compare To Zero1/1 -> Product1/1
  Compare To Zero/1 -> Product/1
  heating/1 -> Product1/2, Compare To Zero1/1, Compare To Zero/1, Product/2
  Product/1 -> Bus Assignment1/14
  Product1/1 -> Bus Assignment1/13

== system carnotUIBK/room_node/EMPTY ==
  note: EMPTY
  sum([S]) : Inport
  AIB_initialize : Subsystem
  BDB_initialize : Subsystem
  Bus Assignment : BusAssignment  AssignedSignals=Ts,Tc,Tr,x_H2O,x_CO2,x_VOC,rho,cp,p
  Bus Assignment1 : BusAssignment  AssignedSignals=Qdot_T_opaque,Qdot_T_ground,Qdot_T_neighbour,Qdot_T_window,Qdot_V_mech,Qdot_V_window,Qdot_V_infiltration,Qdot_S,Qdot_I_person,Qdot_I_light,Qdot_I_electricity,Qdot_H,Qdot_C
  CO2 : carnot/Load/General/Repeating_Profile  period=temperature_timevalues(end)  rep_seq_t=temperature_timevalues(1:end-1)  rep_seq_d=temperature_timeduration  rep_seq_y=temperature_CO2
      settings: SourceProductName=Carnot
  Demux2 : Demux  Outputs=19
      settings: DisplayOption=none
  Gain : Gain  Gain=1e-6*1.529
  Ground1 : Ground
  Ground2 : Ground
  RelHum2x : carnot/Basic/Material_Properties/RelHum2x
      settings: SourceProductName=Carnot
  Sensitive room temperature : Subsystem  mask(SENSITIVE TEMPERATURE){share_c=50}
      mask prompts: share_c "SHARE of convective part, [0,100%]:"
      mask help:
      | This block merges the convective and radiative zone node temperature to the SENSITIVE ZONE TEMPERATURE (weighted arithmetic average of both components).
      |
      | [T] = [Tc; Tr]:  temperature vector of node, °C
      | Ts:              sensitive zone temperature, °C
      mask init: same as carnotUIBK/room_node/2-node/Sensitive room temperature
  Tc : carnot/Load/General/Repeating_Profile  period=temperature_timevalues(end)  rep_seq_t=temperature_timevalues(1:end-1)  rep_seq_d=temperature_timeduration  rep_seq_y=temperature_Tc
      settings: SourceProductName=Carnot
  Terminator{1..7} (7 alike) : Terminator
  Tr : carnot/Load/General/Repeating_Profile  period=temperature_timevalues(end)  rep_seq_t=temperature_timevalues(1:end-1)  rep_seq_d=temperature_timeduration  rep_seq_y=temperature_Tr
      settings: SourceProductName=Carnot
  VOC : carnot/Load/General/Repeating_Profile  period=temperature_timevalues(end)  rep_seq_t=temperature_timevalues(1:end-1)  rep_seq_d=temperature_timeduration  rep_seq_y=temperature_VOC
      settings: SourceProductName=Carnot
  cp0 : Constant  Value=1.0068e+3
  p : carnot/Load/General/Repeating_Profile  period=temperature_timevalues(end)  rep_seq_t=temperature_timevalues(1:end-1)  rep_seq_d=temperature_timeduration  rep_seq_y=temperature_p
      settings: SourceProductName=Carnot
  rH : carnot/Load/General/Repeating_Profile  period=temperature_timevalues(end)  rep_seq_t=temperature_timevalues(1:end-1)  rep_seq_d=temperature_timeduration  rep_seq_y=temperature_rH
      settings: SourceProductName=Carnot
  rho0 : Constant  Value=1.1893
  BDB : Outport  VectorParamsAs1DForOutWhenUnconnected=off
  AIB : Outport  Port=2  VectorParamsAs1DForOutWhenUnconnected=off
  Qdot_sol : Outport  Port=3  VectorParamsAs1DForOutWhenUnconnected=off
  wires:
  Ground2/1 -> Qdot_sol/1
  cp0/1 -> Bus Assignment/9  "cp"
  rho0/1 -> Bus Assignment/8  "rho"
  p/1 -> Bus Assignment/10, RelHum2x/2  "p"
  VOC/1 -> Bus Assignment/7  "x_VOC"
  Tc/1 -> RelHum2x/1, Bus Assignment/3, Sensitive room temperature/2(Tc)  "Tc"
  Tr/1 -> Bus Assignment/4, Sensitive room temperature/1(Tr)  "Tr"
  RelHum2x/1 -> Bus Assignment/5  "x_H2O"
  Gain/1 -> Bus Assignment/6  "x_CO2"
  Sensitive room temperature/1(Ts) -> Bus Assignment/2  "Ts"
  Demux2/7 -> Bus Assignment1/9  "Qdot_S"
  Demux2/8 -> Bus Assignment1/2  "Qdot_T_opaque"
  Demux2/9 -> Bus Assignment1/3  "Qdot_T_ground"
  Demux2/10 -> Bus Assignment1/4  "Qdot_T_neighbour"
  Demux2/11 -> Bus Assignment1/5  "Qdot_T_window"
  Demux2/12 -> Bus Assignment1/6  "Qdot_V_mech"
  Demux2/13 -> Bus Assignment1/7  "Qdot_V_window"
  Demux2/14 -> Bus Assignment1/8  "Qdot_V_infiltration"
  Demux2/15 -> Bus Assignment1/10  "Qdot_I_person"
  Demux2/16 -> Bus Assignment1/11  "Qdot_I_light"
  Demux2/17 -> Bus Assignment1/12  "Qdot_I_electricity"
  Demux2/18 -> Bus Assignment1/13  "Qdot_H"
  Demux2/19 -> Bus Assignment1/14  "Qdot_C"
  Demux2/6 -> Terminator1/1
  Demux2/3 -> Terminator4/1
  Demux2/4 -> Terminator3/1
  Demux2/5 -> Terminator2/1
  Demux2/2 -> Terminator5/1
  Demux2/1 -> Terminator6/1
  rH/1 -> RelHum2x/3
  CO2/1 -> Gain/1
  Bus Assignment/1 -> AIB/1
  AIB_initialize/1(AIB) -> Bus Assignment/1
  BDB_initialize/1(BDB) -> Bus Assignment1/1
  Bus Assignment1/1 -> BDB/1
  Ground1/1 -> Demux2/1
  sum([S])/1 -> Terminator7/1
